simulink subsystem "MCU"  (R2023a)
settings: Solver=VariableStepAuto  StartTime=0.0  StopTime=10.0  RelTol=1e-3
settings Model: Creator=ycheb  LastModifiedBy=ycheb

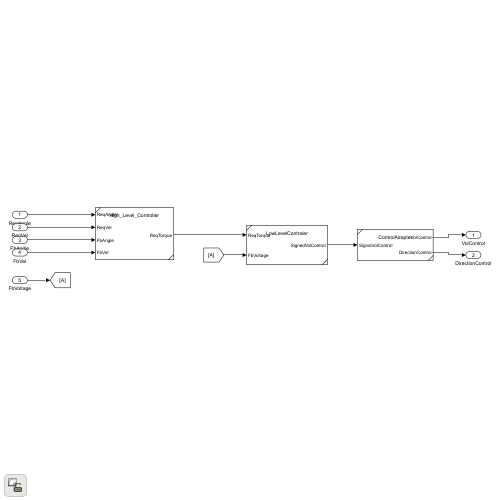
[thumbnail: Simulink's stored preview of the top-level diagram]
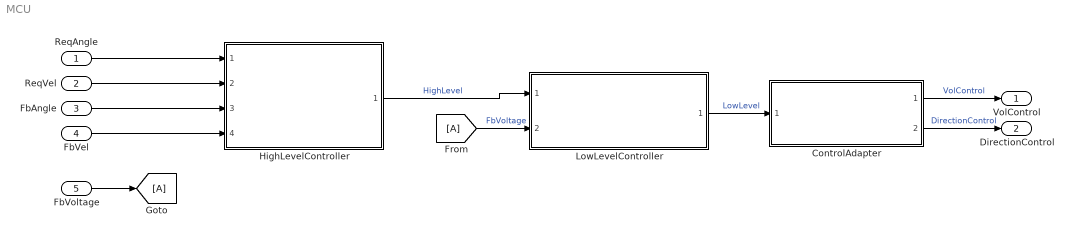
== system MCU ==
  ReqAngle : Inport
  ReqVel : Inport  Port=2
  FbAngle : Inport  Port=3
  FbVel : Inport  Port=4
  FbVoltage : Inport  Port=5
  ControlAdapter : Subsystem  ReferencedSubsystem=ControlAdapter
  From : From
  Goto : Goto
  HighLevelController : Subsystem  ReferencedSubsystem=High_Level_Controller  k_d=k_d  k_p=k_p  k_s=k_s
  LowLevelController : Subsystem  ReferencedSubsystem=LowLevelControler  posled_correc=posled_correc
  VolControl : Outport
  DirectionControl : Outport  Port=2
  wires:
  ControlAdapter/2 -> DirectionControl/1  "DirectionControl"
  HighLevelController/1 -> LowLevelController/1  "HighLevel"
  LowLevelController/1 -> ControlAdapter/1  "LowLevel"
  FbVoltage/1 -> Goto/1
  ReqVel/1 -> HighLevelController/2
  FbAngle/1 -> HighLevelController/3
  ControlAdapter/1 -> VolControl/1  "VolControl"
  ReqAngle/1 -> HighLevelController/1
  FbVel/1 -> HighLevelController/4
  From/1 -> LowLevelController/2  "FbVoltage"
